simulink model "cosim_top"  (R2025b)
settings: Solver=ode4  StartTime=0.0  StopTime=180  FixedStep=0.001  RelTol=1e-3
values from neighbouring files (symbols this model uses):
  eta_mguk = 0.90    (= 0.9)    [create_cosim_top.m]    (also in create_vehicle_model.m; validate_standalone.m)
  K_mguk_torque = 0.8    [create_cosim_top.m]    (also in create_vehicle_model.m)
  k_turbo = 1.5e-5    (= 1.5e-05)    [create_cosim_top.m]    (also in create_vehicle_model.m; validate_standalone.m)
  P_max_mguh = 50e3    (= 50000)    [create_cosim_top.m]    (also in create_vehicle_model.m; validate_standalone.m)
  P_max_mguk = 120e3    (= 120000)    [create_cosim_top.m]    (also in create_vehicle_model.m; validate_standalone.m)
  Q_max_battery = 4e6    (= 4000000)    [create_cosim_top.m]    (also in create_vehicle_model.m)
  SoC_inicial = 0.70    (= 0.7)    [create_cosim_top.m]    (also in create_vehicle_model.m)
  T_volta = 60    [create_cosim_top.m]    (also in create_vehicle_model.m; validate_standalone.m)
  Ts = 1e-3    (= 0.001)    [create_cosim_top.m]    (also in create_vehicle_model.m)
  V_bus_nominal = 400    [create_cosim_top.m]    (also in create_vehicle_model.m)
libraries: simulink x3
settings Model: Creator=Rafael  LastModifiedBy=Rafael

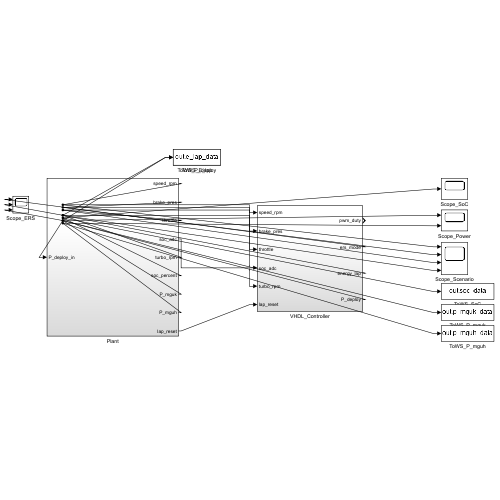
[thumbnail: Simulink's stored preview of the top-level diagram]
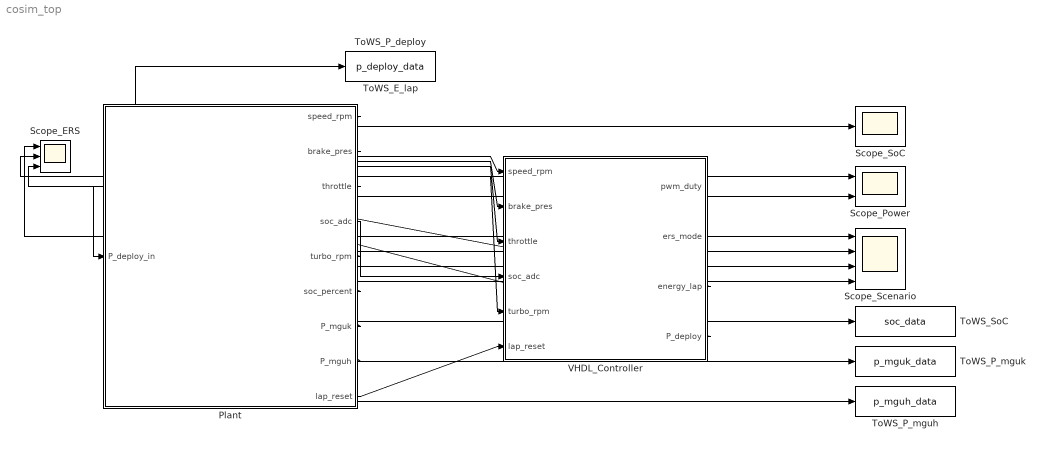
== system cosim_top ==
  Plant : Subsystem
  Scope_ERS : Scope  NumInputPorts=3
  Scope_Power : Scope  NumInputPorts=2
  Scope_Scenario : Scope  NumInputPorts=4
  Scope_SoC : Scope
  ToWS_E_lap : ToWorkspace  VariableName=e_lap_data  SaveFormat=Timeseries  SampleTime=-1
  ToWS_P_deploy : ToWorkspace  VariableName=p_deploy_data  SaveFormat=Timeseries  SampleTime=-1
  ToWS_P_mguh : ToWorkspace  VariableName=p_mguh_data  SaveFormat=Timeseries  SampleTime=-1
  ToWS_P_mguk : ToWorkspace  VariableName=p_mguk_data  SaveFormat=Timeseries  SampleTime=-1
  ToWS_SoC : ToWorkspace  VariableName=soc_data  SaveFormat=Timeseries  SampleTime=-1
  VHDL_Controller : Subsystem
  wires:
  Plant/1(speed_rpm) -> VHDL_Controller/1(speed_rpm), Scope_Scenario/1
  Plant/2(brake_pres) -> VHDL_Controller/2(brake_pres), Scope_Scenario/2
  Plant/3(throttle) -> VHDL_Controller/3(throttle), Scope_Scenario/3
  Plant/4(soc_adc) -> VHDL_Controller/4(soc_adc)
  Plant/5(turbo_rpm) -> VHDL_Controller/5(turbo_rpm), Scope_Scenario/4
  Plant/9(lap_reset) -> VHDL_Controller/6(lap_reset)
  VHDL_Controller/4(P_deploy) -> Plant/1(P_deploy_in), Scope_ERS/3, ToWS_P_deploy/1
  Plant/6(soc_percent) -> Scope_SoC/1, ToWS_SoC/1
  Plant/7(P_mguk) -> Scope_Power/1, ToWS_P_mguk/1
  Plant/8(P_mguh) -> Scope_Power/2, ToWS_P_mguh/1
  VHDL_Controller/2(ers_mode) -> Scope_ERS/1
  VHDL_Controller/3(energy_lap) -> Scope_ERS/2, ToWS_E_lap/1

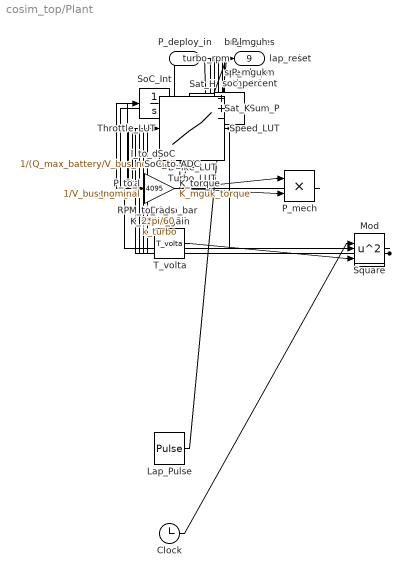
== system cosim_top/Plant ==
  P_deploy_in : Inport
  ADC_to_bar : Gain  Gain=100/4095
  Brake_LUT : Lookup_n-D  NumberOfTableDimensions=1  BreakpointsForDimension1=[0,10,20,28,30,33,36,40,50,60]  Table=[0,0,0,0,3500,4095,2000,0,0,0]  InternalRulePriority=Speed  RndMeth=Simplest
  Clock : Clock
  Eta : Gain  Gain=eta_mguk
  I_to_dSoC : Gain  Gain=1/(Q_max_battery/V_bus_nominal)
  K_torque : Gain  Gain=K_mguk_torque
  K_turbo_gain : Gain  Gain=k_turbo
  Lap_Pulse : DiscretePulseGenerator  Period=T_volta/Ts  SampleTime=Ts
  Mod : Math  Operator=mod
  P_mech : Product
  P_to_I : Gain  Gain=1/V_bus_nominal
  RPM_to_rads : Gain  Gain=2*pi/60
  Sat_H : Saturate  UpperLimit=P_max_mguh  LowerLimit=0
  Sat_K : Saturate  UpperLimit=P_max_mguk  LowerLimit=0
  SoC_Int : Integrator  InitialCondition=SoC_inicial  LimitOutput=on  UpperSaturationLimit=0.95  LowerSaturationLimit=0.20
  SoC_to_ADC : Gain  Gain=4095
  Speed_LUT : Lookup_n-D  NumberOfTableDimensions=1  BreakpointsForDimension1=[0,10,20,28,32,35,38,45,55,60]  Table=[3000,15000,18000,18000,8000,5000,5000,8000,15000,3000]  InternalRulePriority=Speed  RndMeth=Simplest
  Square : Math  Operator=square
  Sum_P : Sum  Inputs=++-
  T_volta : Constant  Value=T_volta
  Throttle_LUT : Lookup_n-D  NumberOfTableDimensions=1  BreakpointsForDimension1=[0,10,20,28,30,35,38,45,55,60]  Table=[2048,3500,4095,4095,0,0,500,2500,4095,2048]  InternalRulePriority=Speed  RndMeth=Simplest
  Turbo_LUT : Lookup_n-D  NumberOfTableDimensions=1  BreakpointsForDimension1=[0,10,20,28,32,36,40,45,55,60]  Table=[20000,45000,60000,65000,30000,20000,25000,40000,60000,20000]  InternalRulePriority=Speed  RndMeth=Simplest
  speed_rpm : Outport
  brake_pres : Outport  Port=2
  throttle : Outport  Port=3
  soc_adc : Outport  Port=4
  turbo_rpm : Outport  Port=5
  soc_percent : Outport  Port=6
  P_mguk : Outport  Port=7
  P_mguh : Outport  Port=8
  lap_reset : Outport  Port=9
  wires:
  Clock/1 -> Mod/1
  T_volta/1 -> Mod/2
  Mod/1 -> Speed_LUT/1, Brake_LUT/1, Throttle_LUT/1, Turbo_LUT/1
  Brake_LUT/1 -> ADC_to_bar/1, brake_pres/1
  Speed_LUT/1 -> RPM_to_rads/1, speed_rpm/1
  ADC_to_bar/1 -> K_torque/1
  K_torque/1 -> P_mech/1
  RPM_to_rads/1 -> P_mech/2
  P_mech/1 -> Eta/1
  Eta/1 -> Sat_K/1
  Turbo_LUT/1 -> Square/1, turbo_rpm/1
  Square/1 -> K_turbo_gain/1
  K_turbo_gain/1 -> Sat_H/1
  Sat_K/1 -> Sum_P/1, P_mguk/1
  Sat_H/1 -> Sum_P/2, P_mguh/1
  P_deploy_in/1 -> Sum_P/3
  Sum_P/1 -> P_to_I/1
  P_to_I/1 -> I_to_dSoC/1
  I_to_dSoC/1 -> SoC_Int/1
  SoC_Int/1 -> SoC_to_ADC/1, soc_percent/1
  Throttle_LUT/1 -> throttle/1
  SoC_to_ADC/1 -> soc_adc/1
  Lap_Pulse/1 -> lap_reset/1

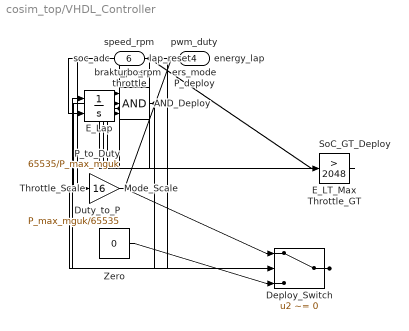
== system cosim_top/VHDL_Controller ==
  speed_rpm : Inport
  brake_pres : Inport  Port=2
  throttle : Inport  Port=3
  soc_adc : Inport  Port=4
  turbo_rpm : Inport  Port=5
  lap_reset : Inport  Port=6
  AND_Deploy : Logic  Inputs=3  AllPortsSameDT=off  OutDataTypeStr=boolean
  Deploy_Switch : Switch  Criteria=u2 ~= 0  SaturateOnIntegerOverflow=off  InputSameDT=off
  Duty_to_P : Gain  Gain=P_max_mguk/65535
  E_LT_Max : simulink/Logic and Bit Operations/Compare To Constant  relop=<  const=4e6  OutDataTypeStr=boolean
  E_Lap : Integrator  ExternalReset=rising
  Mode_Scale : Gain  Gain=3
  P_to_Duty : Gain  Gain=65535/P_max_mguk
  SoC_GT_Deploy : simulink/Logic and Bit Operations/Compare To Constant  relop=>  const=1024  OutDataTypeStr=boolean
  Throttle_GT : simulink/Logic and Bit Operations/Compare To Constant  relop=>  const=2048  OutDataTypeStr=boolean
  Throttle_Scale : Gain  Gain=16
  Zero : Constant  Value=0
  pwm_duty : Outport
  ers_mode : Outport  Port=2
  energy_lap : Outport  Port=3
  P_deploy : Outport  Port=4
  wires:
  throttle/1 -> Throttle_GT/1, Throttle_Scale/1
  soc_adc/1 -> SoC_GT_Deploy/1
  Throttle_Scale/1 -> Duty_to_P/1
  E_Lap/1 -> E_LT_Max/1, energy_lap/1
  Throttle_GT/1 -> AND_Deploy/1
  SoC_GT_Deploy/1 -> AND_Deploy/2
  E_LT_Max/1 -> AND_Deploy/3
  Duty_to_P/1 -> Deploy_Switch/1
  AND_Deploy/1 -> Deploy_Switch/2, Mode_Scale/1
  Zero/1 -> Deploy_Switch/3
  Deploy_Switch/1 -> E_Lap/1, P_to_Duty/1, P_deploy/1
  lap_reset/1 -> E_Lap/2
  P_to_Duty/1 -> pwm_duty/1
  Mode_Scale/1 -> ers_mode/1
